simulink model "Re_q_aero2_2dof_lqi"  (R2025a)
settings: Solver=ode1  StartTime=0.0  StopTime=90  FixedStep=0.002  RelTol=1e-3  EnableMultiTasking=on
values from neighbouring files (symbols this model uses):
  K = lqr(A, B, Q, R)    [aero2_2dof_control_lqi.m]
undefined symbols (not defined in the file or in its folder): HIL, qc_get_step_size
libraries: quarc_library x6, simulink_extras x4, eeGeneralControl x1
settings Model: SimulationMode=external  ExtModeTrigDuration=15000  Creator=MLevis  LastModifiedBy=khanh
settings SolverCC: AlgebraicLoopSolver=TrustRegion  PositivePriorityOrder=on
settings DataIOCC: LimitDataPoints=on  SaveFormat=Array  ReturnWorkspaceOutputs=off
settings DebuggingCC: SolverPrmCheckMsg=warning  UnconnectedInputMsg=warning  UnconnectedOutputMsg=warning  UnconnectedLineMsg=warning  SFUnexpectedBacktrackingDiag=warning  SFNoUnconditionalDefaultTransitionDiag=warning  SFExecutionAtInitializationDiag=none  ArithmeticOperatorsInVariantConditions=warning
settings ModelReferenceCC: EnableRefExpFcnMdlSchedulingChecks=on  PropagateSignalLabelsOutOfModel=off
settings SFSimCC: SimUseLocalCustomCode=off  CustomCodeUndefinedFunction=UseInterfaceOnly
settings RTWCC: SystemTargetFile=quarc_win64.tlc  TemplateMakefile=quarc_default_tmf  RTWUseLocalCustomCode=off  Toolchain=QUARC win64 | nmake (64-bit Windows)  BuildConfiguration=Faster Runs  GPUComputeCapability=3.5  DLArmComputeVersion=19.05  Description=QUARC Win64 Target Using Toolchain
settings CodeAppCC: StateflowObjectComments=on
settings STFCustomTargetCC: SystemTargetFile=quarc_win64.tlc  MultiwordLength=2048.0  DynamicStringBufferSize=256.0  ConcurrentExecutionCompliant=on  UseToolchainInfoCompliant=on
settings GRTTargetCC: ExtMode=on  ExtModeMexFile=quarc_comm  TargetLangStandard=C89/C90 (ANSI)  ParMdlRefBuildCompliant=off  CompOptLevelCompliant=off  CombineOutputUpdateFcns=off  MatFileLogging=off  CPPClassGenCompliant=off  GRTInterface=on
settings ConfigComp: CovMetricSettings=dw  CovSaveCumulativeToWorkspaceVar=on  CovSaveSingleToWorkspaceVar=on  CovExternalEMLEnable=off  CovSFcnEnable=off

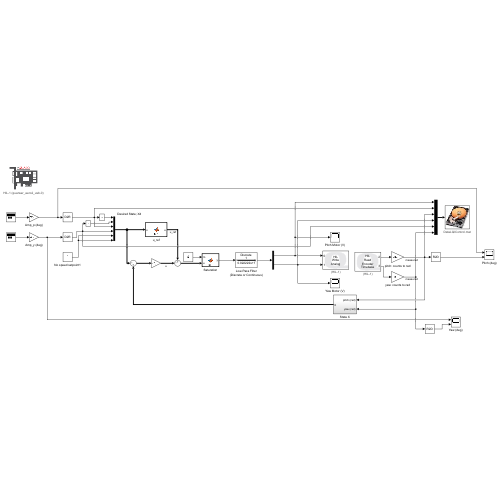
[thumbnail: Simulink's stored preview of the top-level diagram]
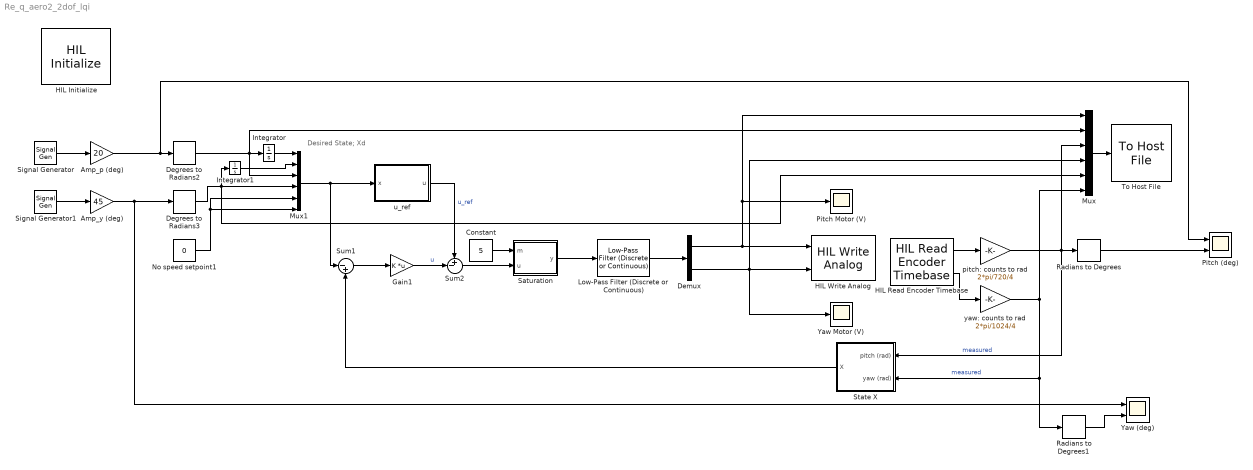
== system Re_q_aero2_2dof_lqi ==
  note: Desired State; Xd
  Amp_p (deg) : Gain  Gain=20
  Amp_y (deg) : Gain  Gain=45
  Constant : Constant  Value=5
  Degrees to Radians2 : simulink_extras/Transformations/Degrees to Radians
  Degrees to Radians3 : simulink_extras/Transformations/Degrees to Radians
  Demux : Demux  Outputs=2
  Gain1 : Gain  Gain=K  Multiplication=Matrix(K*u)
  HIL Initialize : quarc_library/Data Acquisition/Generic/Configuration/HIL Initialize  Priority=-99  object_name=HIL-1  board_type=quanser_aero2_usb  board_number=0  board_options=""  exclusive=off  active=off  hardware_clocks=[0]  clock_modes=[]  initial_clock_frequencies=[]  set_clock_params_at_start=off  set_clock_params_at_switch_in=off  set_clock_frequencies_at_start=off  set_clock_frequencies_at_switch_in=off  analog_input_channels=[0:1]  analog_input_configurations=[]  analog_input_maximums=3  analog_input_minimums=-3  set_analog_input_params_at_start=off  set_analog_input_params_at_switch_in=off  analog_output_channels=[0:1]  analog_output_maximums=24  analog_output_minimums=-24  initial_analog_outputs=[0]  final_analog_outputs=[0]  watchdog_analog_outputs=[0]  set_analog_output_params_at_start=off  set_analog_output_params_at_switch_in=off  set_analog_outputs_at_start=on  set_analog_outputs_at_switch_in=off  set_analog_outputs_at_terminate=on  set_analog_outputs_at_switch_out=off  set_analog_outputs_on_watchdog=on  digital_input_channels=[]  digital_output_channels=[0:1]  digital_output_configuration=[]  initial_digital_outputs=[1]  final_digital_outputs=[0]  watchdog_digital_outputs=[0]  set_digital_output_params_at_start=off  set_digital_output_params_at_switch_in=off  set_digital_outputs_at_start=on  set_digital_outputs_at_switch_in=off  set_digital_outputs_at_terminate=on  set_digital_outputs_at_switch_out=off  set_digital_outputs_on_watchdog=on  encoder_channels=[0:3]  quadrature=[4]  encoder_filter_frequency=[]  initial_encoder_counts=[0]  set_encoder_params_at_start=off  set_encoder_params_at_switch_in=off  set_encoder_counts_at_start=on  set_encoder_counts_at_switch_in=off  pwm_channels=[]  pwm_modes=[]  pwm_frequency=[]  pwm_configuration=[]  pwm_alignment=[]  pwm_polarity=[]  pwm_leading_deadband=[]  pwm_trailing_deadband=[]  initial_pwm_outputs=[]  final_pwm_outputs=[]  watchdog_pwm_outputs=[]  set_pwm_params_at_start=off  set_pwm_params_at_switch_in=off  set_pwm_outputs_at_start=off  set_pwm_outputs_at_switch_in=off  set_pwm_outputs_at_terminate=off  set_pwm_outputs_at_switch_out=off  set_pwm_outputs_on_watchdog=off  other_output_channels=[11000:11002]  initial_other_outputs=[0 1 0]  final_other_outputs=[1 0 0]  watchdog_other_outputs=[0 0 1]  set_other_outputs_at_start=on  set_other_outputs_at_switch_in=off  set_other_outputs_at_terminate=on  set_other_outputs_at_switch_out=off  set_other_outputs_on_watchdog=on
  HIL Read Encoder Timebase : quarc_library/Data Acquisition/Generic/Timebases/HIL Read Encoder Timebase  object_name=HIL-1  clock=0  channels=[2,3]  active=on  vector_output=off  data_type_mode=Inherit via back propagation  data_type=double  overflow_mode=Error on overflow  samples_in_buffer=max(ceil(1/qc_get_step_size), 1)
  HIL Write Analog : quarc_library/Data Acquisition/Generic/Immediate I//O/HIL Write Analog  object_name=HIL-1  channels=[0:1]  sample_time=-1  active=off  vector_input=off
  Integrator : Integrator
  Integrator1 : Integrator
  Low-Pass Filter (Discrete or Continuous) : eeGeneralControl/Low-Pass Filter (Discrete or Continuous)  K=1  T=1/45  B=inf  A=-inf  init_option=Inherited from block input  x0=0  Ts=-1
  Mux : Mux  Inputs=6
  Mux1 : Mux  Inputs=6
  No speed setpoint1 : Constant  Value=0
  Pitch (deg) : Scope  NumInputPorts=2
      settings: TimeSpan=30  ActiveDisplayYMinimum=-38.671875  ActiveDisplayYMaximum=43.046875  DataLoggingVariableName=Aero2_LQR_HW_Pitch
  Pitch Motor (V) : Scope
      settings: TimeSpan=30  ActiveDisplayYMinimum=-30.029954168670933  ActiveDisplayYMaximum=30.034104468469685  DataLoggingVariableName=Aero2_LQR_HW_Vp
  Radians to Degrees : simulink_extras/Transformations/Radians to Degrees
  Radians to Degrees1 : simulink_extras/Transformations/Radians to Degrees
  Saturation : MATLAB Function  TreatAsAtomicUnit=on
  Signal Generator : SignalGenerator  WaveForm=square  Frequency=0.05
  Signal Generator1 : SignalGenerator  WaveForm=square  Frequency=0.04
  State X : Subsystem
  Sum1 : Sum  Inputs=|-+
  Sum2 : Sum  Inputs=+-|
  To Host File : quarc_library/Sinks/To Host/To Host File  source=Specify via dialog (do not evaluate)  file_name=DataLQIControl.mat  variable_name=DataLQIControl  decimation=1  sample_time=-1  file_format=MAT-file v.4  options=No header or footer  append=off  final_file_name=DataLQIControl.mat  encoding=Default  bitrate=2000000
  Yaw (deg) : Scope  NumInputPorts=2
      settings: TimeSpan=30  ActiveDisplayYMinimum=-56.568603515625  ActiveDisplayYMaximum=56.480712890625  DataLoggingVariableName=Aero2_LQR_HW_Yaw
  Yaw Motor (V) : Scope
      settings: TimeSpan=30  ActiveDisplayYMinimum=-30.034648502515605  ActiveDisplayYMaximum=30.034671409288737  DataLoggingVariableName=Aero2_LQR_HW_Vy
  pitch: counts to rad : Gain  Gain=2*pi/720/4
  u_ref : MATLAB Function  TreatAsAtomicUnit=on
  yaw: counts to rad : Gain  Gain=2*pi/1024/4
  wires:
  Signal Generator/1 -> Amp_p (deg)/1
  Amp_p (deg)/1 -> Degrees to Radians2/1, Pitch (deg)/1
  Signal Generator1/1 -> Amp_y (deg)/1
  Amp_y (deg)/1 -> Degrees to Radians3/1, Yaw (deg)/1
  HIL Read Encoder Timebase/2 -> yaw: counts to rad/1
  HIL Read Encoder Timebase/1 -> pitch: counts to rad/1
  pitch: counts to rad/1 -> State X/1(pitch (rad)), Mux/3, Radians to Degrees/1  "measured"
  yaw: counts to rad/1 -> Mux/6, State X/2(yaw (rad)), Radians to Degrees1/1  "measured"
  Radians to Degrees/1 -> Pitch (deg)/2
  Radians to Degrees1/1 -> Yaw (deg)/2
  Mux/1 -> To Host File/1
  Gain1/1 -> Sum2/2  "u"
  Sum2/1 -> Saturation/2(u)
  u_ref/1(u) -> Sum2/1  "u_ref"
  Mux1/1 -> u_ref/1(x), Sum1/1
  Constant/1 -> Saturation/1(m)
  Sum1/1 -> Gain1/1
  Degrees to Radians3/1 -> Mux1/4, Mux/5, Integrator1/1
  Degrees to Radians2/1 -> Mux/2, Mux1/3, Integrator/1
  Integrator/1 -> Mux1/1
  No speed setpoint1/1 -> Mux1/5, Mux1/6
  Integrator1/1 -> Mux1/2
  Demux/1 -> Pitch Motor (V)/1, Mux/1, HIL Write Analog/1
  Demux/2 -> Mux/4, Yaw Motor (V)/1, HIL Write Analog/2
  State X/1(X) -> Sum1/2
  Saturation/1(y) -> Low-Pass Filter (Discrete or Continuous)/1
  Low-Pass Filter (Discrete or Continuous)/1 -> Demux/1

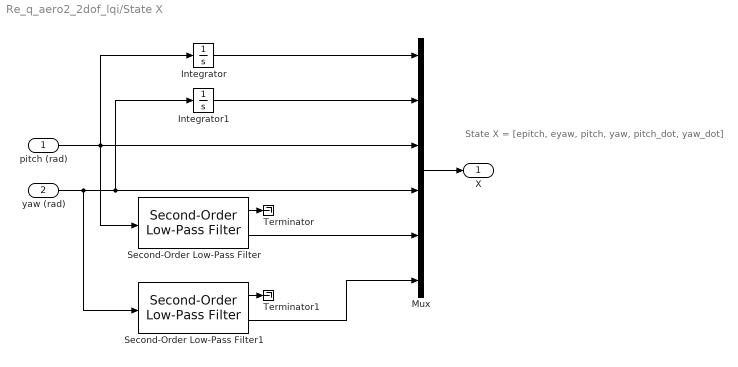
== system Re_q_aero2_2dof_lqi/State X ==
  note: State X = [epitch, eyaw, pitch, yaw, pitch_dot, yaw_dot]
  pitch (rad) : Inport
  yaw (rad) : Inport  Port=2
  Integrator : Integrator
  Integrator1 : Integrator
  Mux : Mux  Inputs=6
  Second-Order Low-Pass Filter : quarc_library/Continuous/Second-Order Low-Pass Filter  params_source=Internal (dialog parameters)  input_width=50  input_zeta=0.8  input_init=0
  Second-Order Low-Pass Filter1 : quarc_library/Continuous/Second-Order Low-Pass Filter  params_source=Internal (dialog parameters)  input_width=50  input_zeta=0.8  input_init=0
  Terminator : Terminator
  Terminator1 : Terminator
  X : Outport
  wires:
  Mux/1 -> X/1
  yaw (rad)/1 -> Integrator1/1, Mux/4, Second-Order Low-Pass Filter1/1
  pitch (rad)/1 -> Second-Order Low-Pass Filter/1, Integrator/1, Mux/3
  Second-Order Low-Pass Filter/2 -> Mux/5
  Second-Order Low-Pass Filter1/2 -> Mux/6
  Second-Order Low-Pass Filter/1 -> Terminator/1
  Second-Order Low-Pass Filter1/1 -> Terminator1/1
  Integrator/1 -> Mux/1
  Integrator1/1 -> Mux/2

== matlab function Re_q_aero2_2dof_lqi/u_ref ==
  data: x input; u output
function u = fcn(x)

Dt = 0.16743; 
% total aero body mass (kg)
Mb = 1.07; 
% distance from aero body plane to center of mass below (m)
Dm = 2.4e-3; 
% Moment of inertia about pitch-axis (kg-m^2)
Jp = 23188500.45 / 1000 * 0.001^2; % from CAD: 23188500.45 g-mm^2
% Moment of inertia about pitch-axis (kg-m^2)
Jy = 23810415.95 / 1000 * 0.001^2; % from CAD: 23810415.95 g-mm^2;
% Gravity (m/s^2)
g = 9.81;
% Stiffness (N-m/V)
Ksp = 0.00744;
% Damping (N-m/V)
Dp = 0.00199;
% Pitch thrust gain (N/V)
Kpp = 0.00321;
% Pitch from yaw thrust gain (N/V)
Kpy = 0.00137;
% Damping (N-m/V)
Dy = 0.00192;
% Thrust (N-m/V)
Kyy = 0.00610;
% Yaw from pitch thrust gain (N/V)
Kyp = -0.00319;

A = [0 0 1 0 0 0;
     0 0 0 1 0 0;
     0 0 0 0 1 0;
     0 0 0 0 0 1;
     0 0 -Ksp/Jp 0 -Dp/Jp 0;
     0 0 0 0 0 -Dy/Jy];
B = [0 0; 0 0; 0 0; 0 0; Kpp*Dt/Jp Kpy*Dt/Jp; Kyp*Dt/Jy Kyy*Dt/Jy];
y = -A*x;
u = B\y;

== matlab function Re_q_aero2_2dof_lqi/Saturation ==
  data: m input; u input; y output
function y = fcn(m,u)
    u_min = -24;
    u_max = 24;
y = ((u_min + u_max) + ...
         u_min .* tanh((u_min - u)*m) + ...
         u_max .* tanh((u - u_max)* m) + ...
         u .* (tanh((u - u_min)*m) - tanh((u - u_max)*m)))./2;
